simulink model "design_of_module"  (R2016a)
settings: Solver=VariableStepAuto  StartTime=0.0  StopTime=4  RelTol=1e-3
libraries: powerlib x24, simulink x1
settings Model: Creator=lenovo  LastModifiedBy=丑是事实
settings SolverCC: ZeroCrossAlgorithm=Adaptive
settings DataIOCC: LimitDataPoints=on
settings DebuggingCC: AllowSymbolicDim=off
settings ModelReferenceCC: PropagateSignalLabelsOutOfModel=off
settings GRTTargetCC: GeneratePreprocessorConditionals=Use local settings

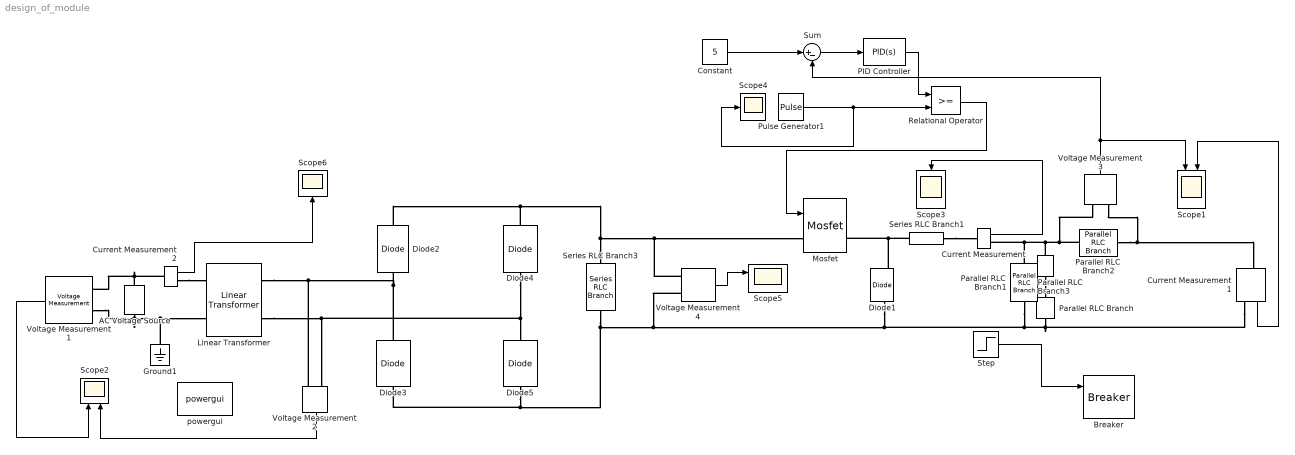
== system design_of_module ==
  AC Voltage Source : powerlib/Electrical Sources/AC Voltage Source  Amplitude=311  Phase=0  Frequency=50  SampleTime=0  Measurements=None  BusType=swing  Pref=10e3  Qref=0  Qmin=-inf  Qmax=+inf
  Breaker : powerlib/Elements/Breaker  InitialState=0  SwitchingTimes="[1/60  5/60]"  External=on  BreakerResistance=5  SnubberResistance=5  SnubberCapacitance=inf  Measurements=None  MoreParameters=on  NoBreakLoop=off
  Constant : Constant  Value=5
  Current Measurement : powerlib/Measurements/Current Measurement  PhasorSimulation=off  OutputType=Complex  PSBequivalent=0
  Current Measurement1 : powerlib/Measurements/Current Measurement  PhasorSimulation=off  OutputType=Complex  PSBequivalent=0
  Current Measurement2 : powerlib/Measurements/Current Measurement  PhasorSimulation=off  OutputType=Complex  PSBequivalent=0
  Diode1 : powerlib/Power Electronics/Diode  Ron=0.001  Lon=0  Vf=0.8  IC=0  UseSnubber=off  Rs=500  Cs=250e-9  Measurements=on
  Diode{2..5} (4 alike) : powerlib/Power Electronics/Diode  Ron=0.001  Lon=0  Vf=0.8  IC=0  UseSnubber=off  Rs=5  Cs=250e-9  Measurements=off
  Ground1 : powerlib/Elements/Ground  LConnTagsString=a
  Linear Transformer : powerlib/Elements/Linear Transformer  UNITS=pu  NominalPower=[ 10e3 50 ]  winding1="[ 220  0  0 ]"  winding2="[ 10  0 0 ]"  ThreeWindings=off  winding3=[ 5e3 0.002 0.08 ]  RmLm=[ 500 500 ]  Measurements=None  DataType=off
  Mosfet : powerlib/Power Electronics/Mosfet  Ron=0.1  Lon=0  Rd=0.01  Vfd=0  IC=0  Rs=1e5  Cs=inf  Measurements=on
  PID Controller : simulink/Continuous/PID Controller  Controller=PID  TimeDomain=Continuous-time  SampleTime=-1  IntegratorMethod=Forward Euler  FilterMethod=Forward Euler  Form=Parallel  UseFilter=on  ControllerParametersSource=internal  P=5000  I=2  D=0.4  N=100  InitialConditionSource=internal  InitialConditionForIntegrator=0  InitialConditionForFilter=0  ExternalReset=none  LimitOutput=off  UpperSaturationLimit=inf  LowerSaturationLimit=-inf  LinearizeAsGain=on  AntiWindupMode=none  Kb=1  TrackingMode=off  Kt=1  PParamMin=[]  PParamMax=[]  IParamMin=[]  IParamMax=[]  DParamMin=[]  DParamMax=[]  NParamMin=[]  NParamMax=[]  KbParamMin=[]  KbParamMax=[]  KtParamMin=[]  KtParamMax=[]  POutMin=[]  POutMax=[]  IOutMin=[]  IOutMax=[]  DOutMin=[]  DOutMax=[]  NOutMin=[]  NOutMax=[]  KbOutMin=[]  KbOutMax=[]  KtOutMin=[]  KtOutMax=[]  IntegratorOutMin=[]  IntegratorOutMax=[]  FilterOutMin=[]  FilterOutMax=[]  SumOutMin=[]  SumOutMax=[]  SumI1OutMin=[]  SumI1OutMax=[]  SumI2OutMin=[]  SumI2OutMax=[]  SumI3OutMin=[]  SumI3OutMax=[]  SumDOutMin=[]  SumDOutMax=[]  SaturationOutMin=[]  SaturationOutMax=[]  IntegratorContinuousStateAttributes=''  IntegratorStateMustResolveToSignalObject=off  IntegratorRTWStateStorageClass=Auto  FilterContinuousStateAttributes=''  FilterStateMustResolveToSignalObject=off  FilterRTWStateStorageClass=Auto  DifferentiatorICPrevScaledInput=0  DifferentiatorOutMin=[]  DifferentiatorOutMax=[]
  Parallel RLC Branch : powerlib/Elements/Parallel RLC Branch  LConnTagsString=a  RConnTagsString=__new0  BranchType=C  Resistance=5  Inductance=1e-3  SetiL0=off  InitialCurrent=0  Capacitance=100e-5  Setx0=off  InitialVoltage=0  Measurements=None
  Parallel RLC Branch1 : powerlib/Elements/Parallel RLC Branch  LConnTagsString=a  RConnTagsString=__new0  BranchType=R  Resistance=2  Inductance=1e-3  SetiL0=off  InitialCurrent=0  Capacitance=7e-4  Setx0=off  InitialVoltage=0  Measurements=None
  Parallel RLC Branch2 : powerlib/Elements/Parallel RLC Branch  LConnTagsString=a  RConnTagsString=__new0  BranchType=R  Resistance=5  Inductance=1e-3  SetiL0=off  InitialCurrent=0  Capacitance=7e-4  Setx0=off  InitialVoltage=0  Measurements=None
  Parallel RLC Branch3 : powerlib/Elements/Parallel RLC Branch  LConnTagsString=a  RConnTagsString=__new0  BranchType=R  Resistance=10  Inductance=1e-3  SetiL0=off  InitialCurrent=0  Capacitance=7e-4  Setx0=off  InitialVoltage=0  Measurements=None
  Pulse Generator1 : DiscretePulseGenerator  PulseType=Time based  Period=0.0001  PulseWidth=50  PhaseDelay=0.000025
  Relational Operator : RelationalOperator  OutDataTypeStr=boolean
  Scope1 : Scope  NumInputPorts=2
  Scope2 : Scope  NumInputPorts=2
  Scope3 : Scope
  Scope4 : Scope
  Scope5 : Scope  NumInputPorts=2
  Scope6 : Scope
  Series RLC Branch1 : powerlib/Elements/Series RLC Branch  LConnTagsString=__new0  RConnTagsString=__new0  BranchType=L  Resistance=2  Inductance=200e-3  SetiL0=off  InitialCurrent=0  Capacitance=1e-6  Setx0=off  InitialVoltage=0  Measurements=None
  Series RLC Branch3 : powerlib/Elements/Series RLC Branch  LConnTagsString=__new0  RConnTagsString=__new0  BranchType=C  Resistance=1  Inductance=1e-3  SetiL0=off  InitialCurrent=0  Capacitance=2200e-6  Setx0=off  InitialVoltage=0  Measurements=None
  Step : Step  SampleTime=0
  Sum : Sum  Inputs=|+-
  Voltage Measurement{1..4} (4 alike) : powerlib/Measurements/Voltage Measurement  PhasorSimulation=off  OutputType=Complex  PSBequivalent=0
  powergui : powerlib/powergui  Priority=1  SimulationMode=Continuous  SolverType=Tustin/Backward Euler (TBE)  SampleTime=50e-6  frequency=60  SPID=off  DisableSnubberDevices=off  DisableRonSwitches=off  DisableVfSwitches=off  SwTol=0  DisplayEquations=off  Interpol=off  ExternalGateDelay=off  methode=off  Ts=10  FunctionMessages=off  echomessages=off  HookPort=off  EnableUseOfTLC=off  x0status=blocks  frequencyindice=0  Pbase=100e6  ErrMax=1e-4  Iterations=50  UnitsV=kV  UnitsW=MW  buscounter=0  RestoreLinks=warning  ResistiveCurrentMeasurement=off  Frange=[0:2:500]  Ylog=off  Xlog=on  ShowGrid=off  save=off  variable=ZData  structure=0  ZoomFFT=off  StartTime=0.0  cycles=1  DisplayStyle=1  fundamental=60  FreqAxis=off  MaxFrequency=1000  frequencyindicesteady=1  RmsSteady=1  display=off
  wires:
  Voltage Measurement1/1 -> Scope2/1
  Voltage Measurement2/1 -> Scope2/2
  Voltage Measurement4/1 -> Scope5/1
  Constant/1 -> Sum/1
  Sum/1 -> PID Controller/1
  PID Controller/1 -> Relational Operator/1
  Relational Operator/1 -> Mosfet/1
  Voltage Measurement3/1 -> Sum/2, Scope1/1
  Current Measurement1/1 -> Scope1/2
  Step/1 -> Breaker/1
  Pulse Generator1/1 -> Scope4/1, Relational Operator/2
  Current Measurement/1 -> Scope3/1
  Current Measurement2/1 -> Scope6/1
  connections:
  Diode3/RConn1 -- Voltage Measurement2/LConn1 -- Linear Transformer/RConn1 -- Diode2/LConn1
  Series RLC Branch3/LConn1 -- Diode2/RConn1 -- Diode4/RConn1 -- Mosfet/LConn1 -- Voltage Measurement4/LConn1
  AC Voltage Source/LConn1 -- Voltage Measurement1/LConn2 -- Linear Transformer/LConn2 -- Ground1/LConn1
  Diode1/RConn1 -- Mosfet/RConn1 -- Series RLC Branch1/LConn1
  Series RLC Branch1/RConn1 -- Current Measurement/LConn1
  Diode4/LConn1 -- Diode5/RConn1 -- Voltage Measurement2/LConn2 -- Linear Transformer/RConn2
  Voltage Measurement3/LConn1 -- Parallel RLC Branch3/LConn1 -- Parallel RLC Branch1/LConn1 -- Current Measurement/RConn1 -- Parallel RLC Branch2/LConn1
  Voltage Measurement3/LConn2 -- Parallel RLC Branch2/RConn1 -- Current Measurement1/LConn1
  Diode5/LConn1 -- Diode3/LConn1 -- Voltage Measurement4/LConn2 -- Current Measurement1/RConn1 -- Parallel RLC Branch/RConn1 -- Parallel RLC Branch1/RConn1 -- Diode1/LConn1 -- Series RLC Branch3/RConn1
  Current Measurement2/LConn1 -- AC Voltage Source/RConn1 -- Voltage Measurement1/LConn1
  Parallel RLC Branch3/RConn1 -- Parallel RLC Branch/LConn1
  Current Measurement2/RConn1 -- Linear Transformer/LConn1
